simulink model "mex4"  (R2022b)
settings: Solver=VariableStepAuto  StartTime=0.0  StopTime=20  RelTol=1e-3
settings Model: Creator=PJ  LastModifiedBy=PJ

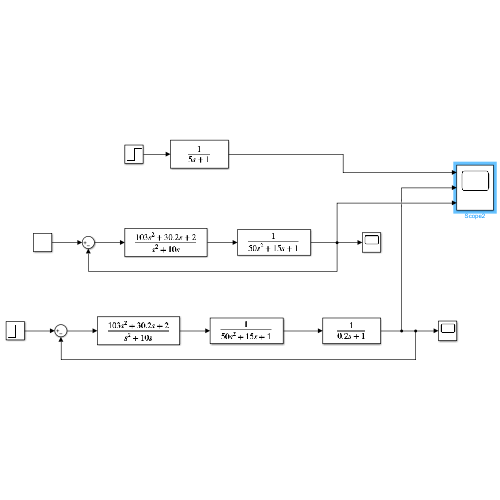
[thumbnail: Simulink's stored preview of the top-level diagram]
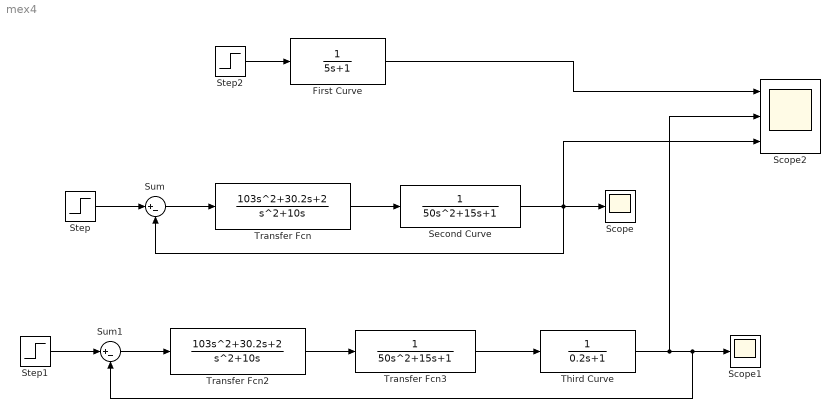
== system mex4 ==
  First Curve : TransferFcn  Denominator=[5 1]
  Scope : Scope
  Scope1 : Scope
  Scope2 : Scope  NumInputPorts=3
  Second Curve : TransferFcn  Denominator=[50 15 1]
  Step : Step  SampleTime=0
  Step1 : Step  SampleTime=0
  Step2 : Step  SampleTime=0
  Sum : Sum  Inputs=|+-
  Sum1 : Sum  Inputs=|+-
  Third Curve : TransferFcn  Denominator=[0.2 1]
  Transfer Fcn : TransferFcn  Numerator=[103 30.2 2]  Denominator=[1 10 0]
  Transfer Fcn2 : TransferFcn  Numerator=[103 30.2 2]  Denominator=[1 10 0]
  Transfer Fcn3 : TransferFcn  Denominator=[50 15 1]
  wires:
  Transfer Fcn/1 -> Second Curve/1
  Second Curve/1 -> Sum/2, Scope2/3, Scope/1
  Sum/1 -> Transfer Fcn/1
  Step/1 -> Sum/1
  Transfer Fcn2/1 -> Transfer Fcn3/1
  Sum1/1 -> Transfer Fcn2/1
  Step1/1 -> Sum1/1
  Transfer Fcn3/1 -> Third Curve/1
  Third Curve/1 -> Scope2/2, Sum1/2, Scope1/1
  Step2/1 -> First Curve/1
  First Curve/1 -> Scope2/1
